simulink model "exampleModel_bus_axi_w_4ptavg"  (R2017b)
settings: Solver=VariableStepAuto  StartTime=0.0  StopTime=10e-5  RelTol=1e-3
PreLoadFcn:
  | setup
values from neighbouring files (symbols this model uses):
  axiClk = 156.25e6    (= 156250000)    [setup.m]    (also in setup_exampleModel_bus_axi_simulink.m; setup_exampleModel_bus_axi_simulink_lcls2.m; setup_lcls2_pcav.m; sysgen_signal.m)
  cav1p1_addr = 204    [setup_exampleModel_bus_axi_simulink.m]    (also in setup_exampleModel_bus_axi_simulink_lcls2.m; setup_lcls2_pcav.m; sysgen_signal.m)
  cav1p2_addr = cav1p1_addr * 2    (= 408)    [setup_exampleModel_bus_axi_simulink.m]    (also in setup_exampleModel_bus_axi_simulink_lcls2.m; setup_lcls2_pcav.m; sysgen_signal.m)
  cav2p1_addr = cav1p1_addr * 3    (= 612)    [setup_exampleModel_bus_axi_simulink.m]    (also in setup_exampleModel_bus_axi_simulink_lcls2.m; setup_lcls2_pcav.m; sysgen_signal.m)
  cav2p2_addr = cav1p1_addr * 4    (= 816)    [setup_exampleModel_bus_axi_simulink.m]    (also in setup_exampleModel_bus_axi_simulink_lcls2.m; setup_lcls2_pcav.m; sysgen_signal.m)
  Fadc = Fs/interleavedChannels    (= 29750000)    [setup.m]    (also in setup_exampleModel_bus_axi_simulink.m = 357000000; setup_exampleModel_bus_axi_simulink_lcls2.m = 351000000; setup_lcls2_pcav.m = 357000000; sysgen_signal.m = 357000000)
  fir_lpf = fir1(15, w_lpf)    [setup_exampleModel_bus_axi_simulink.m]    (also in setup_exampleModel_bus_axi_simulink_lcls2.m; setup_lcls2_pcav.m)
  Fproc = 204e6    (= 204000000)    [setup_exampleModel_bus_axi_simulink.m]    (also in setup_exampleModel_bus_axi_simulink_lcls2.m = 200571400; setup_lcls2_pcav.m; sysgen_signal.m)
  Fsig = Fproc/12    (= 17000000)    [setup_exampleModel_bus_axi_simulink.m]    (also in setup_exampleModel_bus_axi_simulink_lcls2.m = 16714283.3333; setup_lcls2_pcav.m)
  Tadc = 1/fadc    (= 2.80112044818e-09)    [cavity_signal.m]    (also in setup_exampleModel_bus_axi_simulink.m; setup_exampleModel_bus_axi_simulink_lcls2.m = 2.849002849e-09; setup_lcls2_pcav.m; setup_pcav_simulink.m)
undefined symbols (not defined in the file or in its folder): AXI4, Lite
libraries: xbsIndex_r4 x2870, llrf_lib x10, simulink x3
(part 10 of 15)

== system exampleModel_bus_axi_w_4ptavg/example/dsp/Cav2/c1p2_windowing_func3 ==
  imag : Inport
  real : Inport  Port=2
  eval_window : Inport  Port=3
  "CORDIC 6.0 " : xbsIndex_r4/CORDIC 6.0   functional_selection=Translate  architectural_configuration=Parallel  pipelining_mode=Maximum  data_format=SignedFraction  phase_format=Scaled_Radians  input_width=18  output_width=18  round_mode=Truncate  iterations=0  precision=0  compensation_scaling=No_Scale_Compensation  coarse_rotation=on  aclken=off  aresetn=off  out_tready=off  cartesian_has_tuser=off  cartesian_has_tlast=off  cartesian_tuser_width=1  phase_has_tuser=off  phase_has_tlast=off  phase_tuser_width=1  out_tlast_behv=Null  flow_control=NonBlocking  optimize_goal=Resources  trim_axipin_name=on  simulation_type=hybrid_sim  simulation_model=sysgen:cordic_v6_0  data_path_portlist={'s_axis_cartesian_tdata_imag', 's_axis_cartesian_tdata_real', 's_axis_phase_tdata_phase', 'm_axis_dout_tdata_imag', 'm_axis_dout_tdata_real', 'm_axis_dout_tdata_phase','m_axis_dout_tdata'}  ip_name=CORDIC  ip_version=6.0  dsptool_ready=true  ipcore_usecache=true  ipcore_useipmodelcache=true  wrapper_available=true  port_translation_map={ 'aclken' => 'en', 'aresetn' => 'rst' }  block_type=cordic_v6_0
      settings: infoedit=CORDIC 6.0
  Gateway Out{1..5,7} (6 alike) : xbsIndex_r4/Gateway Out  inherit_from_input=off  hdl_port=off  rows=1  columns=1  UseAsDAC=off  DACChannel='1'  interface=None  automatic_assignment=on  address_offset=hex2dec('00')  intf_name=''  intf_description=''  timing_constraint=None  locs_specified=off  LOCs={}  io_standard={}  block_type=gatewayout
  Scope{1..4} (4 alike) : Scope  NumInputPorts=3
  four_point_avg : Subsystem
  Window_profile : Outport
  wires:
  four_point_avg/1(Out1) -> Gateway Out2/1, Window_profile/1
  "CORDIC 6.0 "/3 -> Gateway Out4/1, Gateway Out1/1, four_point_avg/1(In1)
  [cav1_p2_dc_tvalid] -> "CORDIC 6.0 "/1
  imag/1 -> "CORDIC 6.0 "/2
  real/1 -> "CORDIC 6.0 "/3
  Gateway Out5/1 -> Scope3/1, Scope2/2
  Gateway Out7/1 -> Scope4/2, Scope3/2
  [c1p2_pt_cntr] -> Gateway Out7/1
  eval_window/1 -> [window]
  "CORDIC 6.0 "/2 -> Gateway Out5/1
  Gateway Out4/1 -> Scope4/1, Scope2/1
  Gateway Out1/1 -> Scope1/1
  Gateway Out2/1 -> Scope1/2
  [window] -> Gateway Out3/1
  Gateway Out3/1 -> Scope4/3

== system exampleModel_bus_axi_w_4ptavg/example/dsp/Cav2/c2p1_Masking_window1 ==
  note: delay for the comparison because Axilite register
      | takes a about 40 dsp clk cycles to load in
  phi_reset_trig : Inport
  start_pt : Inport  Port=2
  stop_pt : Inport  Port=3
  delay_amt : Inport  Port=4
  delay_latch : Inport  Port=5
  AddSub1 : xbsIndex_r4/AddSub  mode=Addition  use_carryin=off  use_carryout=off  en=off  latency=1  precision=User Defined  arith_type=Unsigned  n_bits=16  bin_pt=0  quantization=Truncate  overflow=Wrap  use_behavioral_HDL=off  hw_selection=Fabric  pipelined=off  dbl_ovrd=off  block_type=addsub
  AddSub4 : xbsIndex_r4/AddSub  mode=Addition  use_carryin=off  use_carryout=off  en=on  latency=1  precision=User Defined  arith_type=Unsigned  n_bits=16  bin_pt=0  quantization=Truncate  overflow=Saturate  use_behavioral_HDL=off  hw_selection=Fabric  pipelined=off  dbl_ovrd=off  block_type=addsub
  Constant1 : xbsIndex_r4/Constant  const=40  gui_display_data_type=Fixed-point  arith_type=Unsigned  n_bits=16  bin_pt=0  preci_type=Single  exp_width=8  frac_width=24  explicit_period=off  period=1  equ=P=C  opselect=C  inp2=PCIN>>17  opr=+  inp1=P  carry=CIN  dbl_ovrd=off  block_type=constant
  Constant11 : xbsIndex_r4/Constant  const=55  gui_display_data_type=Fixed-point  arith_type=Unsigned  n_bits=16  bin_pt=0  preci_type=Single  exp_width=8  frac_width=24  explicit_period=off  period=1  equ=P=C  opselect=C  inp2=PCIN>>17  opr=+  inp1=P  carry=CIN  dbl_ovrd=off  block_type=constant
  Constant2 : xbsIndex_r4/Constant  const=106  gui_display_data_type=Fixed-point  arith_type=Unsigned  n_bits=16  bin_pt=0  preci_type=Single  exp_width=8  frac_width=24  explicit_period=off  period=1  equ=P=C  opselect=C  inp2=PCIN>>17  opr=+  inp1=P  carry=CIN  dbl_ovrd=off  block_type=constant
  Constant3 : xbsIndex_r4/Constant  const=87  gui_display_data_type=Fixed-point  arith_type=Unsigned  n_bits=16  bin_pt=0  preci_type=Single  exp_width=8  frac_width=24  explicit_period=off  period=1  equ=P=C  opselect=C  inp2=PCIN>>17  opr=+  inp1=P  carry=CIN  dbl_ovrd=off  block_type=constant
  Convert{1,4..5,7..8} (5 alike) : xbsIndex_r4/Convert  gui_display_data_type=Boolean  arith_type=Boolean  n_bits=1  bin_pt=0  float_type=Single  exp_bits=8  fraction_bits=24  quantization=Truncate  overflow=Wrap  en=off  latency=1  pipeline=off  dbl_ovrd=off  block_type=convert
  Convert11 : xbsIndex_r4/Convert  gui_display_data_type=Fixed-point  arith_type=Unsigned  n_bits=1  bin_pt=0  float_type=Single  exp_bits=8  fraction_bits=24  quantization=Truncate  overflow=Wrap  en=off  latency=1  pipeline=off  dbl_ovrd=off  block_type=convert
  Convert2 : xbsIndex_r4/Convert  gui_display_data_type=Fixed-point  arith_type=Unsigned  n_bits=1  bin_pt=0  float_type=Single  exp_bits=8  fraction_bits=24  quantization=Truncate  overflow=Wrap  en=off  latency=1  pipeline=off  dbl_ovrd=off  block_type=convert
  Convert3 : xbsIndex_r4/Convert  gui_display_data_type=Boolean  arith_type=Boolean  n_bits=16  bin_pt=14  float_type=Single  exp_bits=8  fraction_bits=24  quantization=Truncate  overflow=Wrap  en=off  latency=1  pipeline=off  dbl_ovrd=off  block_type=convert
  Convert6 : xbsIndex_r4/Convert  gui_display_data_type=Fixed-point  arith_type=Unsigned  n_bits=8  bin_pt=0  float_type=Single  exp_bits=8  fraction_bits=24  quantization=Truncate  overflow=Saturate  en=off  latency=1  pipeline=off  dbl_ovrd=off  block_type=convert
  Counter : xbsIndex_r4/Counter  cnt_type=Count Limited  cnt_to=(2^15)  operation=Up  start_count=0  cnt_by_val=1  arith_type=Unsigned  n_bits=16  bin_pt=0  load_pin=off  rst=on  en=on  explicit_period=on  period=12/Fproc  use_behavioral_HDL=off  implementation=Fabric  dbl_ovrd=off  block_type=counter
  Delay{,1..4,6..7} (7 alike) : xbsIndex_r4/Delay  rst=off  infoeditControl=Selection of Reset will increase slice count due to use of real FFs and instead of SRLs  en=off  latency=1  reg_retiming=off  dbl_ovrd=off  block_type=delay
  Delay5 : xbsIndex_r4/Delay  rst=off  infoeditControl=Selection of Reset will increase slice count due to use of real FFs and instead of SRLs  en=off  latency=3  reg_retiming=off  dbl_ovrd=off  block_type=delay
  Display1 : Display
  Down Sample1 : xbsIndex_r4/Down Sample  sample_ratio=12  sample_phase="Last Value of Frame  (most efficient)"  en=off  rst=off  latency=1  dbl_ovrd=off  block_type=dsamp
  Down Sample2 : xbsIndex_r4/Down Sample  sample_ratio=12  sample_phase="Last Value of Frame  (most efficient)"  en=off  rst=off  latency=1  dbl_ovrd=off  block_type=dsamp
  Gateway Out{1..3,5,27..29} (7 alike) : xbsIndex_r4/Gateway Out  inherit_from_input=off  hdl_port=on  rows=1  columns=1  UseAsDAC=off  DACChannel='1'  interface=None  automatic_assignment=on  address_offset=hex2dec('00')  intf_name=''  intf_description=''  timing_constraint=None  locs_specified=off  LOCs={}  io_standard={}  block_type=gatewayout
  Gateway Out16 : xbsIndex_r4/Gateway Out  inherit_from_input=off  hdl_port=off  rows=1  columns=1  UseAsDAC=off  DACChannel='1'  interface=None  automatic_assignment=on  address_offset=hex2dec('00')  intf_name=''  intf_description=''  timing_constraint=None  locs_specified=off  LOCs={}  io_standard={}  block_type=gatewayout
  Gateway Out17 : xbsIndex_r4/Gateway Out  inherit_from_input=off  hdl_port=off  rows=1  columns=1  UseAsDAC=off  DACChannel='1'  interface=None  automatic_assignment=on  address_offset=hex2dec('00')  intf_name=''  intf_description=''  timing_constraint=None  locs_specified=off  LOCs={}  io_standard={}  block_type=gatewayout
  Gateway Out18 : xbsIndex_r4/Gateway Out  inherit_from_input=off  hdl_port=off  rows=1  columns=1  UseAsDAC=off  DACChannel='1'  interface=None  automatic_assignment=on  address_offset=hex2dec('00')  intf_name=''  intf_description=''  timing_constraint=None  locs_specified=off  LOCs={}  io_standard={}  block_type=gatewayout
  Logical1 : xbsIndex_r4/Logical  logical_function=AND  inputs=2  en=off  latency=1  precision=Full  arith_type=Unsigned  n_bits=16  bin_pt=0  align_bp=on  dbl_ovrd=off  block_type=logical
  Logical2 : xbsIndex_r4/Logical  logical_function=AND  inputs=2  en=off  latency=1  precision=Full  arith_type=Unsigned  n_bits=16  bin_pt=0  align_bp=on  dbl_ovrd=off  block_type=logical
  Register : xbsIndex_r4/Register  init=44  rst=off  en=on  dbl_ovrd=off  block_type=register
  Register1 : xbsIndex_r4/Register  init=0  rst=off  en=on  dbl_ovrd=off  block_type=register
  Register10 : xbsIndex_r4/Register  init=0  rst=off  en=off  dbl_ovrd=off  block_type=register
  Register5 : xbsIndex_r4/Register  init=0  rst=off  en=off  dbl_ovrd=off  block_type=register
  Register6 : xbsIndex_r4/Register  init=100  rst=off  en=off  dbl_ovrd=off  block_type=register
  Relational1 : xbsIndex_r4/Relational  mode=a<b  op_type=Bool  en=on  latency=1  dbl_ovrd=off  block_type=relational
  Relational2 : xbsIndex_r4/Relational  mode=a>b  op_type=Bool  en=off  latency=1  dbl_ovrd=off  block_type=relational
  Relational3 : xbsIndex_r4/Relational  mode=a<b  op_type=Bool  en=on  latency=1  dbl_ovrd=off  block_type=relational
  Relational4 : xbsIndex_r4/Relational  mode=a>b  op_type=Bool  en=on  latency=1  dbl_ovrd=off  block_type=relational
  Relational5 : xbsIndex_r4/Relational  mode=a<b  op_type=Bool  en=on  latency=1  dbl_ovrd=off  block_type=relational
  Relational6 : xbsIndex_r4/Relational  mode=a>b  op_type=Bool  en=on  latency=1  dbl_ovrd=off  block_type=relational
  Scope1 : Scope  NumInputPorts=3
  Scope10 : Scope  NumInputPorts=3
  Scope2 : Scope  NumInputPorts=2
  Scope5 : Scope  NumInputPorts=3
  counter : Outport
  eval_window : Outport  Port=2
  integral_trig : Outport  Port=3
  flo_window : Outport  Port=4
  delay_val : Outport  Port=5
  wires:
  Gateway Out5/1 -> Scope2/2
  start_pt/1 -> Register5/1
  phi_reset_trig/1 -> Register10/1
  Register5/1 -> Down Sample1/1
  stop_pt/1 -> Register6/1
  Register6/1 -> Down Sample2/1
  Delay2/1 -> Relational4/2
  Delay3/1 -> AddSub1/1, Gateway Out2/1, Relational3/2
  Constant1/1 -> Relational2/2
  Relational3/1 -> Gateway Out28/1, Convert7/1
  Relational4/1 -> Gateway Out27/1, Convert8/1
  Gateway Out28/1 -> Scope10/2
  Gateway Out29/1 -> Scope2/1, Scope10/3
  Gateway Out27/1 -> Scope10/1
  Logical1/1 -> Convert11/1
  Convert8/1 -> Logical1/1
  Convert7/1 -> Gateway Out3/1, Logical1/2
  Convert11/1 -> eval_window/1, Gateway Out29/1
  Convert5/1 -> integral_trig/1, Gateway Out5/1
  Relational5/1 -> Convert5/1
  Relational2/1 -> Relational6/3, Relational1/3, Relational5/3, Relational3/3, Relational4/3
  Counter/1 -> Convert6/1
  Constant11/1 -> AddSub1/2
  AddSub1/1 -> Relational5/2
  Register10/1 -> Convert3/1
  Down Sample1/1 -> Delay2/1
  Down Sample2/1 -> Delay3/1
  Gateway Out1/1 -> Scope1/1
  Gateway Out2/1 -> Scope1/2
  Gateway Out3/1 -> Scope1/3
  Delay1/1 -> Relational4/1
  Delay4/1 -> Relational3/1
  Delay5/1 -> Gateway Out1/1
  Delay7/1 -> Relational1/1
  Constant2/1 -> Relational1/2
  Relational1/1 -> Convert1/1
  Logical2/1 -> Convert2/1
  Convert1/1 -> Logical2/2
  Convert2/1 -> flo_window/1
  Delay6/1 -> Relational6/1
  Constant3/1 -> Relational6/2
  Relational6/1 -> Convert4/1
  Convert4/1 -> Logical2/1
  Gateway Out18/1 -> Scope5/3
  delay_latch/1 -> Gateway Out18/1, Delay/1, AddSub4/3
  Register/1 -> AddSub4/1, delay_val/1, Gateway Out17/1
  Delay/1 -> Register/2
  Gateway Out17/1 -> Scope5/2
  delay_amt/1 -> AddSub4/2, Gateway Out16/1
  Gateway Out16/1 -> Scope5/1, Display1/1
  AddSub4/1 -> Register/1
  Convert3/1 -> Register1/2, Register1/1, Counter/1
  Register1/1 -> Counter/2
  Convert6/1 -> Delay5/1, counter/1, Delay1/1, Delay4/1, Relational2/1, Delay6/1, Delay7/1, Relational5/1

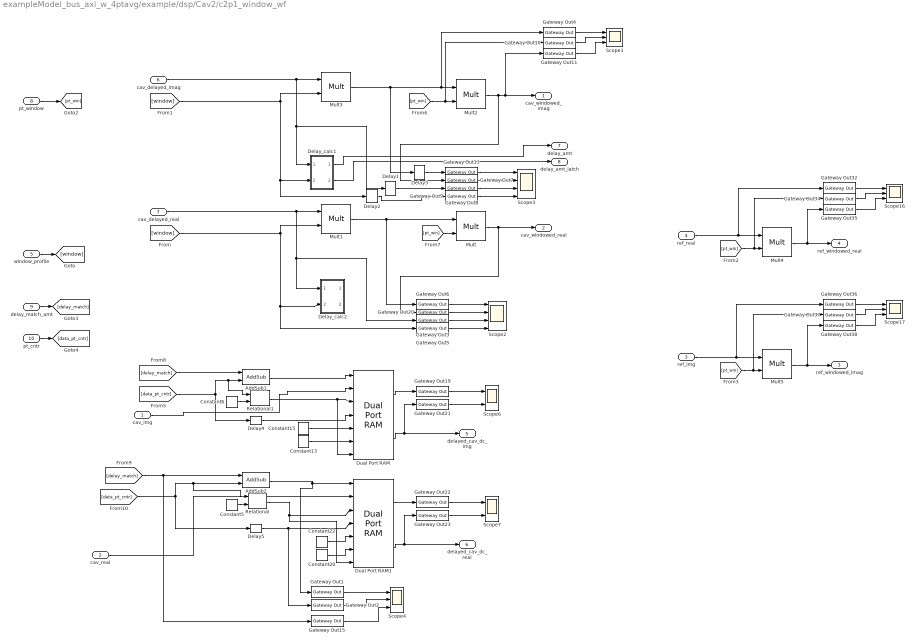
== system exampleModel_bus_axi_w_4ptavg/example/dsp/Cav2/c2p1_window_wf  ==
  cav_img : Inport
  cav_real : Inport  Port=2
  ref_img : Inport  Port=3
  ref_real : Inport  Port=4
  window_profile : Inport  Port=5
  cav_delayed_imag : Inport  Port=6
  cav_delayed_real : Inport  Port=7
  pt_window : Inport  Port=8
  delay_match_amt : Inport  Port=9
  pt_cntr : Inport  Port=10
  AddSub1 : xbsIndex_r4/AddSub  mode=Addition  use_carryin=off  use_carryout=off  en=off  latency=1  precision=User Defined  arith_type=Unsigned  n_bits=16  bin_pt=0  quantization=Truncate  overflow=Wrap  use_behavioral_HDL=off  hw_selection=Fabric  pipelined=off  dbl_ovrd=off  block_type=addsub
  AddSub2 : xbsIndex_r4/AddSub  mode=Addition  use_carryin=off  use_carryout=off  en=off  latency=1  precision=User Defined  arith_type=Unsigned  n_bits=16  bin_pt=0  quantization=Truncate  overflow=Wrap  use_behavioral_HDL=off  hw_selection=Fabric  pipelined=off  dbl_ovrd=off  block_type=addsub
  Constant13 : xbsIndex_r4/Constant  const=1  gui_display_data_type=Boolean  arith_type=Boolean  n_bits=16  bin_pt=14  preci_type=Single  exp_width=8  frac_width=24  explicit_period=off  period=1  equ=P=C  opselect=C  inp2=PCIN>>17  opr=+  inp1=P  carry=CIN  dbl_ovrd=off  block_type=constant
  Constant{5..6,15,22} (4 alike) : xbsIndex_r4/Constant  const=0  gui_display_data_type=Fixed-point  arith_type=Signed (2's comp)  n_bits=18  bin_pt=16  preci_type=Single  exp_width=8  frac_width=24  explicit_period=off  period=1  equ=P=C  opselect=C  inp2=PCIN>>17  opr=+  inp1=P  carry=CIN  dbl_ovrd=off  block_type=constant
  Constant20 : xbsIndex_r4/Constant  const=1  gui_display_data_type=Boolean  arith_type=Boolean  n_bits=16  bin_pt=14  preci_type=Single  exp_width=8  frac_width=24  explicit_period=off  period=1  equ=P=C  opselect=C  inp2=PCIN>>17  opr=+  inp1=P  carry=CIN  dbl_ovrd=off  block_type=constant
  Delay1 : xbsIndex_r4/Delay  rst=off  infoeditControl=Selection of Reset will increase slice count due to use of real FFs and instead of SRLs  en=off  latency=6  reg_retiming=off  dbl_ovrd=off  block_type=delay
  Delay2 : xbsIndex_r4/Delay  rst=off  infoeditControl=Selection of Reset will increase slice count due to use of real FFs and instead of SRLs  en=off  latency=6  reg_retiming=off  dbl_ovrd=off  block_type=delay
  Delay3 : xbsIndex_r4/Delay  rst=off  infoeditControl=Selection of Reset will increase slice count due to use of real FFs and instead of SRLs  en=off  latency=3  reg_retiming=off  dbl_ovrd=off  block_type=delay
  Delay4 : xbsIndex_r4/Delay  rst=off  infoeditControl=Selection of Reset will increase slice count due to use of real FFs and instead of SRLs  en=off  latency=1  reg_retiming=off  dbl_ovrd=off  block_type=delay
  Delay5 : xbsIndex_r4/Delay  rst=off  infoeditControl=Selection of Reset will increase slice count due to use of real FFs and instead of SRLs  en=off  latency=1  reg_retiming=off  dbl_ovrd=off  block_type=delay
  Delay_calc1 : Subsystem
  Delay_calc2 : Subsystem
  Dual Port RAM : xbsIndex_r4/Dual Port RAM  depth=2^16  initVector=zeros(2^16,1)  distributed_mem=Block RAM  init_a=0  init_b=0  rst_a=off  rst_b=off  en_a=off  en_b=on  latency=1  write_mode_A=Read After Write  write_mode_B=Read Before Write  optimize=Area  dbl_ovrd=off  block_type=dpram
  Dual Port RAM1 : xbsIndex_r4/Dual Port RAM  depth=2^16  initVector=zeros(2^16,1)  distributed_mem=Block RAM  init_a=0  init_b=0  rst_a=off  rst_b=off  en_a=off  en_b=on  latency=1  write_mode_A=Read After Write  write_mode_B=Read Before Write  optimize=Area  dbl_ovrd=off  block_type=dpram
  Gateway Out{1..3,5..9,13,15,19..23} (15 alike) : xbsIndex_r4/Gateway Out  inherit_from_input=off  hdl_port=off  rows=1  columns=1  UseAsDAC=off  DACChannel='1'  interface=None  automatic_assignment=on  address_offset=hex2dec('00')  intf_name=''  intf_description=''  timing_constraint=None  locs_specified=off  LOCs={}  io_standard={}  block_type=gatewayout
  Gateway Out{4,10..11,32,34..38} (9 alike) : xbsIndex_r4/Gateway Out  inherit_from_input=off  hdl_port=on  rows=1  columns=1  UseAsDAC=off  DACChannel='1'  interface=None  automatic_assignment=on  address_offset=hex2dec('00')  intf_name=''  intf_description=''  timing_constraint=None  locs_specified=off  LOCs={}  io_standard={}  block_type=gatewayout
  Mult{,2,4..5} (4 alike) : xbsIndex_r4/Mult  precision=User Defined  arith_type="Signed  (2's comp)"  n_bits=18  bin_pt=16  quantization=Truncate  overflow=Wrap  en=off  latency=3  use_behavioral_HDL=off  opt=Speed  use_embedded=on  optimum_pipeline=off  pipeline=on  dbl_ovrd=off  use_rpm=on  placement_style=Triangular  block_type=mult
  Mult1 : xbsIndex_r4/Mult  precision=User Defined  arith_type="Signed  (2's comp)"  n_bits=18  bin_pt=17  quantization=Truncate  overflow=Wrap  en=off  latency=3  use_behavioral_HDL=off  opt=Speed  use_embedded=on  optimum_pipeline=off  pipeline=on  dbl_ovrd=off  use_rpm=on  placement_style=Triangular  block_type=mult
  Mult3 : xbsIndex_r4/Mult  precision=User Defined  arith_type="Signed  (2's comp)"  n_bits=18  bin_pt=17  quantization=Truncate  overflow=Wrap  en=off  latency=3  use_behavioral_HDL=off  opt=Speed  use_embedded=on  optimum_pipeline=off  pipeline=on  dbl_ovrd=off  use_rpm=on  placement_style=Triangular  block_type=mult
  Relational : xbsIndex_r4/Relational  mode=a>b  op_type=Bool  en=off  latency=1  dbl_ovrd=off  block_type=relational
  Relational1 : xbsIndex_r4/Relational  mode=a>b  op_type=Bool  en=off  latency=1  dbl_ovrd=off  block_type=relational
  Scope{1,4,16..17} (4 alike) : Scope  NumInputPorts=3
  Scope2 : Scope  NumInputPorts=4
  Scope3 : Scope  NumInputPorts=4
  Scope6 : Scope  NumInputPorts=2
  Scope7 : Scope  NumInputPorts=2
  cav_windowed_imag : Outport
  cav_windowed_real : Outport  Port=2
  ref_windowed_imag : Outport  Port=3
  ref_windowed_real : Outport  Port=4
  delayed_cav_dc_img : Outport  Port=5
  delayed_cav_dc_real : Outport  Port=6
  delay_amt : Outport  Port=7
  delay_amt_latch : Outport  Port=8
  wires:
  cav_real/1 -> Dual Port RAM1/2
  Relational/1 -> Dual Port RAM1/7, Dual Port RAM1/3
  Mult2/1 -> Gateway Out11/1, cav_windowed_imag/1, Gateway Out7/1
  Gateway Out23/1 -> Scope7/2
  Gateway Out21/1 -> Scope6/2
  Dual Port RAM1/1 -> Gateway Out22/1
  [data_pt_cntr] -> Relational1/1, AddSub1/2, Delay4/1
  Constant15/1 -> Dual Port RAM/5
  Gateway Out20/1 -> Scope2/2
  AddSub1/1 -> Dual Port RAM/1
  [pt_win] -> Gateway Out10/1, Mult2/2
  Gateway Out8/1 -> Scope3/3
  Gateway Out3/1 -> Scope2/3
  Constant13/1 -> Dual Port RAM/6
  Mult/1 -> cav_windowed_real/1, Gateway Out20/1
  cav_delayed_imag/1 -> Mult3/1, Delay_calc1/1(wav), Delay1/1
  [delay_match] -> Gateway Out15/1, AddSub2/1
  Gateway Out19/1 -> Scope6/1
  Gateway Out9/1 -> Scope3/4
  [data_pt_cntr] -> Delay5/1, Relational/1, AddSub2/2
  Dual Port RAM/1 -> Gateway Out19/1
  Gateway Out22/1 -> Scope7/1
  [window] -> Delay_calc1/2(win), Delay2/1, Mult3/2
  [window] -> Mult1/2, Delay_calc2/2(win), Gateway Out5/1
  cav_delayed_real/1 -> Delay_calc2/1(wav), Gateway Out3/1, Mult1/1
  Constant20/1 -> Dual Port RAM1/6
  Mult1/1 -> Gateway Out6/1, Mult/1
  Constant22/1 -> Dual Port RAM1/5
  Gateway Out6/1 -> Scope2/1
  Gateway Out13/1 -> Scope3/1
  [delay_match] -> AddSub1/1
  Gateway Out5/1 -> Scope2/4
  Gateway Out7/1 -> Scope3/2
  [pt_win] -> Mult/2
  Gateway Out35/1 -> Scope16/3
  ref_img/1 -> Gateway Out36/1, Mult5/1
  [pt_win] -> Gateway Out37/1, Mult5/2
  [pt_win] -> Gateway Out34/1, Mult4/2
  ref_real/1 -> Gateway Out32/1, Mult4/1
  Mult5/1 -> ref_windowed_imag/1, Gateway Out38/1
  Gateway Out38/1 -> Scope17/3
  Gateway Out36/1 -> Scope17/1
  Gateway Out32/1 -> Scope16/1
  Gateway Out34/1 -> Scope16/2
  Mult4/1 -> ref_windowed_real/1, Gateway Out35/1
  Gateway Out37/1 -> Scope17/2
  window_profile/1 -> [window]
  Delay_calc1/1(delay_amt) -> delay_amt/1
  pt_window/1 -> [pt_win]
  delay_match_amt/1 -> [delay_match]
  pt_cntr/1 -> [data_pt_cntr]
  Mult3/1 -> Delay3/1, Gateway Out4/1, Mult2/1
  Delay1/1 -> Gateway Out8/1
  Delay2/1 -> Gateway Out9/1
  Delay3/1 -> Gateway Out13/1
  Delay_calc1/2(delay_fb_latch) -> delay_amt_latch/1
  Gateway Out1/1 -> Scope4/1
  Gateway Out2/1 -> Scope4/2
  AddSub2/1 -> Gateway Out1/1, Dual Port RAM1/1
  cav_img/1 -> Dual Port RAM/2
  Delay4/1 -> Dual Port RAM/4
  Gateway Out15/1 -> Scope4/3
  Delay5/1 -> Gateway Out2/1, Dual Port RAM1/4
  Dual Port RAM1/2 -> delayed_cav_dc_real/1, Gateway Out23/1
  Dual Port RAM/2 -> delayed_cav_dc_img/1, Gateway Out21/1
  Constant5/1 -> Relational/2
  Constant6/1 -> Relational1/2
  Relational1/1 -> Dual Port RAM/7, Dual Port RAM/3
  Gateway Out10/1 -> Scope1/2
  Gateway Out4/1 -> Scope1/1
  Gateway Out11/1 -> Scope1/3

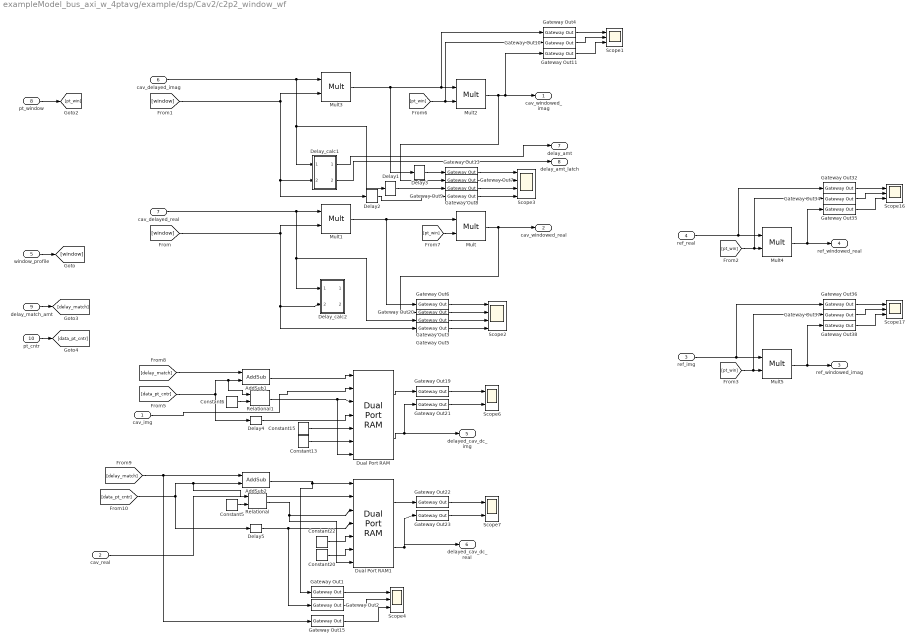
== system exampleModel_bus_axi_w_4ptavg/example/dsp/Cav2/c2p2_window_wf ==
  cav_img : Inport
  cav_real : Inport  Port=2
  ref_img : Inport  Port=3
  ref_real : Inport  Port=4
  window_profile : Inport  Port=5
  cav_delayed_imag : Inport  Port=6
  cav_delayed_real : Inport  Port=7
  pt_window : Inport  Port=8
  delay_match_amt : Inport  Port=9
  pt_cntr : Inport  Port=10
  AddSub1 : xbsIndex_r4/AddSub  mode=Addition  use_carryin=off  use_carryout=off  en=off  latency=1  precision=User Defined  arith_type=Unsigned  n_bits=16  bin_pt=0  quantization=Truncate  overflow=Wrap  use_behavioral_HDL=off  hw_selection=Fabric  pipelined=off  dbl_ovrd=off  block_type=addsub
  AddSub2 : xbsIndex_r4/AddSub  mode=Addition  use_carryin=off  use_carryout=off  en=off  latency=1  precision=User Defined  arith_type=Unsigned  n_bits=16  bin_pt=0  quantization=Truncate  overflow=Wrap  use_behavioral_HDL=off  hw_selection=Fabric  pipelined=off  dbl_ovrd=off  block_type=addsub
  Constant13 : xbsIndex_r4/Constant  const=1  gui_display_data_type=Boolean  arith_type=Boolean  n_bits=16  bin_pt=14  preci_type=Single  exp_width=8  frac_width=24  explicit_period=off  period=1  equ=P=C  opselect=C  inp2=PCIN>>17  opr=+  inp1=P  carry=CIN  dbl_ovrd=off  block_type=constant
  Constant{5..6,15,22} (4 alike) : xbsIndex_r4/Constant  const=0  gui_display_data_type=Fixed-point  arith_type=Signed (2's comp)  n_bits=18  bin_pt=16  preci_type=Single  exp_width=8  frac_width=24  explicit_period=off  period=1  equ=P=C  opselect=C  inp2=PCIN>>17  opr=+  inp1=P  carry=CIN  dbl_ovrd=off  block_type=constant
  Constant20 : xbsIndex_r4/Constant  const=1  gui_display_data_type=Boolean  arith_type=Boolean  n_bits=16  bin_pt=14  preci_type=Single  exp_width=8  frac_width=24  explicit_period=off  period=1  equ=P=C  opselect=C  inp2=PCIN>>17  opr=+  inp1=P  carry=CIN  dbl_ovrd=off  block_type=constant
  Delay1 : xbsIndex_r4/Delay  rst=off  infoeditControl=Selection of Reset will increase slice count due to use of real FFs and instead of SRLs  en=off  latency=6  reg_retiming=off  dbl_ovrd=off  block_type=delay
  Delay2 : xbsIndex_r4/Delay  rst=off  infoeditControl=Selection of Reset will increase slice count due to use of real FFs and instead of SRLs  en=off  latency=6  reg_retiming=off  dbl_ovrd=off  block_type=delay
  Delay3 : xbsIndex_r4/Delay  rst=off  infoeditControl=Selection of Reset will increase slice count due to use of real FFs and instead of SRLs  en=off  latency=3  reg_retiming=off  dbl_ovrd=off  block_type=delay
  Delay4 : xbsIndex_r4/Delay  rst=off  infoeditControl=Selection of Reset will increase slice count due to use of real FFs and instead of SRLs  en=off  latency=1  reg_retiming=off  dbl_ovrd=off  block_type=delay
  Delay5 : xbsIndex_r4/Delay  rst=off  infoeditControl=Selection of Reset will increase slice count due to use of real FFs and instead of SRLs  en=off  latency=1  reg_retiming=off  dbl_ovrd=off  block_type=delay
  Delay_calc1 : Subsystem
  Delay_calc2 : Subsystem
  Dual Port RAM : xbsIndex_r4/Dual Port RAM  depth=2^16  initVector=zeros(2^16,1)  distributed_mem=Block RAM  init_a=0  init_b=0  rst_a=off  rst_b=off  en_a=off  en_b=on  latency=1  write_mode_A=Read After Write  write_mode_B=Read Before Write  optimize=Area  dbl_ovrd=off  block_type=dpram
  Dual Port RAM1 : xbsIndex_r4/Dual Port RAM  depth=2^16  initVector=zeros(2^16,1)  distributed_mem=Block RAM  init_a=0  init_b=0  rst_a=off  rst_b=off  en_a=off  en_b=on  latency=1  write_mode_A=Read After Write  write_mode_B=Read Before Write  optimize=Area  dbl_ovrd=off  block_type=dpram
  Gateway Out{1..3,5..9,13,15,19..23} (15 alike) : xbsIndex_r4/Gateway Out  inherit_from_input=off  hdl_port=off  rows=1  columns=1  UseAsDAC=off  DACChannel='1'  interface=None  automatic_assignment=on  address_offset=hex2dec('00')  intf_name=''  intf_description=''  timing_constraint=None  locs_specified=off  LOCs={}  io_standard={}  block_type=gatewayout
  Gateway Out{4,10..11,32,34..38} (9 alike) : xbsIndex_r4/Gateway Out  inherit_from_input=off  hdl_port=on  rows=1  columns=1  UseAsDAC=off  DACChannel='1'  interface=None  automatic_assignment=on  address_offset=hex2dec('00')  intf_name=''  intf_description=''  timing_constraint=None  locs_specified=off  LOCs={}  io_standard={}  block_type=gatewayout
  Mult{,2,4..5} (4 alike) : xbsIndex_r4/Mult  precision=User Defined  arith_type="Signed  (2's comp)"  n_bits=18  bin_pt=16  quantization=Truncate  overflow=Wrap  en=off  latency=3  use_behavioral_HDL=off  opt=Speed  use_embedded=on  optimum_pipeline=off  pipeline=on  dbl_ovrd=off  use_rpm=on  placement_style=Triangular  block_type=mult
  Mult1 : xbsIndex_r4/Mult  precision=User Defined  arith_type="Signed  (2's comp)"  n_bits=18  bin_pt=17  quantization=Truncate  overflow=Wrap  en=off  latency=3  use_behavioral_HDL=off  opt=Speed  use_embedded=on  optimum_pipeline=off  pipeline=on  dbl_ovrd=off  use_rpm=on  placement_style=Triangular  block_type=mult
  Mult3 : xbsIndex_r4/Mult  precision=User Defined  arith_type="Signed  (2's comp)"  n_bits=18  bin_pt=17  quantization=Truncate  overflow=Wrap  en=off  latency=3  use_behavioral_HDL=off  opt=Speed  use_embedded=on  optimum_pipeline=off  pipeline=on  dbl_ovrd=off  use_rpm=on  placement_style=Triangular  block_type=mult
  Relational : xbsIndex_r4/Relational  mode=a>b  op_type=Bool  en=off  latency=1  dbl_ovrd=off  block_type=relational
  Relational1 : xbsIndex_r4/Relational  mode=a>b  op_type=Bool  en=off  latency=1  dbl_ovrd=off  block_type=relational
  Scope{1,4,16..17} (4 alike) : Scope  NumInputPorts=3
  Scope2 : Scope  NumInputPorts=4
  Scope3 : Scope  NumInputPorts=4
  Scope6 : Scope  NumInputPorts=2
  Scope7 : Scope  NumInputPorts=2
  cav_windowed_imag : Outport
  cav_windowed_real : Outport  Port=2
  ref_windowed_imag : Outport  Port=3
  ref_windowed_real : Outport  Port=4
  delayed_cav_dc_img : Outport  Port=5
  delayed_cav_dc_real : Outport  Port=6
  delay_amt : Outport  Port=7
  delay_amt_latch : Outport  Port=8
  wires:
  cav_real/1 -> Dual Port RAM1/2
  Relational/1 -> Dual Port RAM1/7, Dual Port RAM1/3
  Mult2/1 -> Gateway Out11/1, cav_windowed_imag/1, Gateway Out7/1
  Gateway Out23/1 -> Scope7/2
  Gateway Out21/1 -> Scope6/2
  Dual Port RAM1/1 -> Gateway Out22/1
  [data_pt_cntr] -> Relational1/1, AddSub1/2, Delay4/1
  Constant15/1 -> Dual Port RAM/5
  Gateway Out20/1 -> Scope2/2
  AddSub1/1 -> Dual Port RAM/1
  [pt_win] -> Gateway Out10/1, Mult2/2
  Gateway Out8/1 -> Scope3/3
  Gateway Out3/1 -> Scope2/3
  Constant13/1 -> Dual Port RAM/6
  Mult/1 -> cav_windowed_real/1, Gateway Out20/1
  cav_delayed_imag/1 -> Mult3/1, Delay_calc1/1(wav), Delay1/1
  [delay_match] -> Gateway Out15/1, AddSub2/1
  Gateway Out19/1 -> Scope6/1
  Gateway Out9/1 -> Scope3/4
  [data_pt_cntr] -> Delay5/1, Relational/1, AddSub2/2
  Dual Port RAM/1 -> Gateway Out19/1
  Gateway Out22/1 -> Scope7/1
  [window] -> Delay_calc1/2(win), Delay2/1, Mult3/2
  [window] -> Mult1/2, Delay_calc2/2(win), Gateway Out5/1
  cav_delayed_real/1 -> Delay_calc2/1(wav), Gateway Out3/1, Mult1/1
  Constant20/1 -> Dual Port RAM1/6
  Mult1/1 -> Gateway Out6/1, Mult/1
  Constant22/1 -> Dual Port RAM1/5
  Gateway Out6/1 -> Scope2/1
  Gateway Out13/1 -> Scope3/1
  [delay_match] -> AddSub1/1
  Gateway Out5/1 -> Scope2/4
  Gateway Out7/1 -> Scope3/2
  [pt_win] -> Mult/2
  Gateway Out35/1 -> Scope16/3
  ref_img/1 -> Gateway Out36/1, Mult5/1
  [pt_win] -> Gateway Out37/1, Mult5/2
  [pt_win] -> Gateway Out34/1, Mult4/2
  ref_real/1 -> Gateway Out32/1, Mult4/1
  Mult5/1 -> ref_windowed_imag/1, Gateway Out38/1
  Gateway Out38/1 -> Scope17/3
  Gateway Out36/1 -> Scope17/1
  Gateway Out32/1 -> Scope16/1
  Gateway Out34/1 -> Scope16/2
  Mult4/1 -> ref_windowed_real/1, Gateway Out35/1
  Gateway Out37/1 -> Scope17/2
  window_profile/1 -> [window]
  Delay_calc1/1(delay_amt) -> delay_amt/1
  pt_window/1 -> [pt_win]
  delay_match_amt/1 -> [delay_match]
  pt_cntr/1 -> [data_pt_cntr]
  Mult3/1 -> Delay3/1, Gateway Out4/1, Mult2/1
  Delay1/1 -> Gateway Out8/1
  Delay2/1 -> Gateway Out9/1
  Delay3/1 -> Gateway Out13/1
  Delay_calc1/2(delay_fb_latch) -> delay_amt_latch/1
  Gateway Out1/1 -> Scope4/1
  Gateway Out2/1 -> Scope4/2
  AddSub2/1 -> Gateway Out1/1, Dual Port RAM1/1
  cav_img/1 -> Dual Port RAM/2
  Delay4/1 -> Dual Port RAM/4
  Gateway Out15/1 -> Scope4/3
  Delay5/1 -> Gateway Out2/1, Dual Port RAM1/4
  Dual Port RAM1/2 -> delayed_cav_dc_real/1, Gateway Out23/1
  Dual Port RAM/2 -> delayed_cav_dc_img/1, Gateway Out21/1
  Constant5/1 -> Relational/2
  Constant6/1 -> Relational1/2
  Relational1/1 -> Dual Port RAM/7, Dual Port RAM/3
  Gateway Out10/1 -> Scope1/2
  Gateway Out4/1 -> Scope1/1
  Gateway Out11/1 -> Scope1/3

== system exampleModel_bus_axi_w_4ptavg/example/dsp/Ref/IQ_select ==
  IQ_stream_in : Inport
  IQ_chan_sel : Inport  Port=2
  Bus Creator5 : BusCreator  Inputs=3
  Bus Selector : BusSelector  OutputSignals=ddcI,ddcQ,sync
  Bus Selector3 : BusSelector  OutputSignals=ddcI,ddcQ,ddcSync,ddcChannel
  Channel Select3 : llrf_lib/Sysgen/Single Rate/Channel Select  SystemSampleTime=-1
      settings: SourceProductName=LLRF Library
  ddcI : Outport
  ddcQ : Outport  Port=2
  sync : Outport  Port=3
  wires:
  IQ_stream_in/1 -> Bus Selector3/1
  IQ_chan_sel/1 -> Channel Select3/5
  Channel Select3/3 -> Bus Creator5/3  "sync"
  Bus Selector3/2 -> Channel Select3/2  "<ddcQ>"
  Channel Select3/1 -> Bus Creator5/1  "ddcI"
  Channel Select3/2 -> Bus Creator5/2  "ddcQ"
  Bus Selector3/1 -> Channel Select3/1  "<ddcI>"
  Bus Selector3/4 -> Channel Select3/4  "<ddcChannel>"
  Bus Selector3/3 -> Channel Select3/3  "<ddcSync>"
  Bus Creator5/1 -> Bus Selector/1
  Bus Selector/1 -> ddcI/1  "<ddcI>"
  Bus Selector/2 -> ddcQ/1  "<ddcQ>"
  Bus Selector/3 -> sync/1  "<sync>"

== system exampleModel_bus_axi_w_4ptavg/example/dsp/Ref/PA_select ==
  PA_bus : Inport
  PA_chan_sel : Inport  Port=2
  Bus Selector1 : BusSelector  OutputSignals=amp,phase,sync,channel
  Channel Select1 : llrf_lib/Sysgen/Single Rate/Channel Select  SystemSampleTime=-1
      settings: SourceProductName=LLRF Library
  Amp : Outport
  Phase : Outport  Port=2
  sync : Outport  Port=3
  wires:
  PA_bus/1 -> Bus Selector1/1
  PA_chan_sel/1 -> Channel Select1/5
  Channel Select1/3 -> sync/1  "sync"
  Channel Select1/2 -> Phase/1  "phase"
  Channel Select1/1 -> Amp/1  "amp"
  Bus Selector1/4 -> Channel Select1/4  "<channel>"
  Bus Selector1/3 -> Channel Select1/3  "<sync>"
  Bus Selector1/2 -> Channel Select1/2  "<phase>"
  Bus Selector1/1 -> Channel Select1/1  "<amp>"

== system exampleModel_bus_axi_w_4ptavg/example/dsp/Cav1/DDC NCO1/pulse_catcher ==
  In1 : Inport
  Convert : xbsIndex_r4/Convert  gui_display_data_type=Boolean  arith_type=Boolean  n_bits=16  bin_pt=14  float_type=Single  exp_bits=8  fraction_bits=24  quantization=Truncate  overflow=Wrap  en=off  latency=1  pipeline=off  dbl_ovrd=off  block_type=convert
  Delay : xbsIndex_r4/Delay  rst=off  infoeditControl=Selection of Reset will increase slice count due to use of real FFs and instead of SRLs  en=off  latency=5  reg_retiming=off  dbl_ovrd=off  block_type=delay
  Delay1 : xbsIndex_r4/Delay  rst=off  infoeditControl=Selection of Reset will increase slice count due to use of real FFs and instead of SRLs  en=off  latency=1  reg_retiming=off  dbl_ovrd=off  block_type=delay
  Register : xbsIndex_r4/Register  init=0  rst=on  en=on  dbl_ovrd=off  block_type=register
  Out1 : Outport
  wires:
  In1/1 -> Convert/1, Delay1/1
  Delay/1 -> Register/2
  Register/1 -> Out1/1
  Convert/1 -> Register/3, Delay/1
  Delay1/1 -> Register/1

== system exampleModel_bus_axi_w_4ptavg/example/dsp/Cav1/Subsystem/four_point_avg ==
  In1 : Inport
  AddSub1 : xbsIndex_r4/AddSub  mode=Addition  use_carryin=off  use_carryout=off  en=off  latency=1  precision=User Defined  arith_type="Signed  (2's comp)"  n_bits=33  bin_pt=31  quantization=Truncate  overflow=Saturate  use_behavioral_HDL=off  hw_selection=Fabric  pipelined=off  dbl_ovrd=off  block_type=addsub
  AddSub2 : xbsIndex_r4/AddSub  mode=Addition  use_carryin=off  use_carryout=off  en=off  latency=1  precision=User Defined  arith_type="Signed  (2's comp)"  n_bits=33  bin_pt=31  quantization=Truncate  overflow=Saturate  use_behavioral_HDL=off  hw_selection=Fabric  pipelined=off  dbl_ovrd=off  block_type=addsub
  AddSub3 : xbsIndex_r4/AddSub  mode=Addition  use_carryin=off  use_carryout=off  en=off  latency=1  precision=User Defined  arith_type="Signed  (2's comp)"  n_bits=33  bin_pt=31  quantization=Truncate  overflow=Saturate  use_behavioral_HDL=off  hw_selection=Fabric  pipelined=off  dbl_ovrd=off  block_type=addsub
  CMult{1..4} (4 alike) : xbsIndex_r4/CMult  const=0.25  gui_display_data_type=Fixed-point  const_n_bits=18  const_bin_pt=16  float_type=Single  exp_bits=8  fraction_bits=24  en=off  latency=1  precision=User Defined  arith_type="Signed  (2's comp)"  n_bits=33  bin_pt=31  quantization=Truncate  overflow=Saturate  use_behavioral_HDL=off  mem_type=Distributed RAM  pipeline=off  dbl_ovrd=off  block_type=cmult
  Delay1 : xbsIndex_r4/Delay  rst=off  infoeditControl=Selection of Reset will increase slice count due to use of real FFs and instead of SRLs  en=off  latency=1  reg_retiming=off  dbl_ovrd=off  block_type=delay
  Delay2 : xbsIndex_r4/Delay  rst=off  infoeditControl=Selection of Reset will increase slice count due to use of real FFs and instead of SRLs  en=off  latency=1  reg_retiming=off  dbl_ovrd=off  block_type=delay
  Delay3 : xbsIndex_r4/Delay  rst=off  infoeditControl=Selection of Reset will increase slice count due to use of real FFs and instead of SRLs  en=off  latency=1  reg_retiming=off  dbl_ovrd=off  block_type=delay
  Out1 : Outport
  wires:
  Delay1/1 -> CMult2/1, Delay2/1
  AddSub2/1 -> AddSub3/1
  Delay2/1 -> CMult1/1, Delay3/1
  CMult2/1 -> AddSub1/2
  Delay3/1 -> CMult3/1
  AddSub1/1 -> AddSub3/2
  In1/1 -> CMult4/1, Delay1/1
  CMult3/1 -> AddSub2/2
  AddSub3/1 -> Out1/1
  CMult4/1 -> AddSub1/1
  CMult1/1 -> AddSub2/1

== system exampleModel_bus_axi_w_4ptavg/example/dsp/Cav1/Subsystem/freq_err ==
  note: find ratio with NCO
  note: 2*pi*dt
  note: pi*(scaled_phi))
  note: w = d_phi/dt = (pi*(scaled_phi))/dt
  note: f=w/(2*pi)
  note: window for start/stop evaluating the phase
  raw_phase : Inport
  window : Inport  Port=2
  reset : Inport  Port=3
  AddSub : xbsIndex_r4/AddSub  mode=Addition  use_carryin=off  use_carryout=off  en=on  latency=1  precision=User Defined  arith_type="Signed  (2's comp)"  n_bits=64  bin_pt=32  quantization=Truncate  overflow=Saturate  use_behavioral_HDL=off  hw_selection=Fabric  pipelined=off  dbl_ovrd=off  block_type=addsub
  Constant1 : xbsIndex_r4/Constant  const=-Fsig  gui_display_data_type=Fixed-point  arith_type=Signed (2's comp)  n_bits=26  bin_pt=0  preci_type=Single  exp_width=8  frac_width=24  explicit_period=off  period=1  equ=P=C  opselect=C  inp2=PCIN>>17  opr=+  inp1=P  carry=CIN  dbl_ovrd=off  block_type=constant
  Constant8 : xbsIndex_r4/Constant  const=-Fsig  gui_display_data_type=Fixed-point  arith_type=Signed (2's comp)  n_bits=26  bin_pt=0  preci_type=Single  exp_width=8  frac_width=24  explicit_period=off  period=1  equ=P=C  opselect=C  inp2=PCIN>>17  opr=+  inp1=P  carry=CIN  dbl_ovrd=off  block_type=constant
  Convert : xbsIndex_r4/Convert  gui_display_data_type=Fixed-point  arith_type="Signed  (2's comp)"  n_bits=32  bin_pt=32  float_type=Single  exp_bits=8  fraction_bits=24  quantization=Truncate  overflow=Saturate  en=off  latency=1  pipeline=off  dbl_ovrd=off  block_type=convert
  Convert1 : xbsIndex_r4/Convert  gui_display_data_type=Fixed-point  arith_type="Signed  (2's comp)"  n_bits=32  bin_pt=32  float_type=Single  exp_bits=8  fraction_bits=24  quantization=Truncate  overflow=Saturate  en=off  latency=1  pipeline=off  dbl_ovrd=off  block_type=convert
  Convert3 : xbsIndex_r4/Convert  gui_display_data_type=Boolean  arith_type=Boolean  n_bits=16  bin_pt=14  float_type=Single  exp_bits=8  fraction_bits=24  quantization=Truncate  overflow=Wrap  en=off  latency=1  pipeline=off  dbl_ovrd=off  block_type=convert
  Delay : Delay  DelayLength=3  InitialCondition=0
  Delay1 : Delay  DelayLength=3  InitialCondition=0
  Delay2 : Delay  DelayLength=3  InitialCondition=0
  Delay3 : xbsIndex_r4/Delay  rst=off  infoeditControl=Selection of Reset will increase slice count due to use of real FFs and instead of SRLs  en=off  latency=10  reg_retiming=off  dbl_ovrd=off  block_type=delay
  Delay4 : xbsIndex_r4/Delay  rst=off  infoeditControl=Selection of Reset will increase slice count due to use of real FFs and instead of SRLs  en=off  latency=1  reg_retiming=off  dbl_ovrd=off  block_type=delay
  Delay5 : xbsIndex_r4/Delay  rst=off  infoeditControl=Selection of Reset will increase slice count due to use of real FFs and instead of SRLs  en=off  latency=1  reg_retiming=off  dbl_ovrd=off  block_type=delay
  Display1 : Display
  Display6 : Display
  Display8 : Display
  Divide : xbsIndex_r4/Divide  flow_control=NonBlocking  axi_optimize_goal=Resources  algorithm_type=Radix2  infoedit1=Specify output fraction-width for Fixed-point division.  fractional_width=31  infoedit2=Specify latency for Floating-point division.  latency=1  rate=1  has_a_tlast=off  has_a_tuser=off  has_b_tlast=off  has_b_tuser=off  en=off  has_result_tready=off  result_tlast_behv=Pass_A_TLAST  has_underflow=off  has_overflow=off  has_invalid_op=off  has_divide_by_zero=off  fpo_op_type=mergeddivide  block_type=divide
      settings: infoedit=Blocking: Wait for data on all inputs, allow back-pressure.<br>NonBlocking: operate every cycle in which all inputs are valid, no back-pressure.
  Divide1 : xbsIndex_r4/Divide  flow_control=NonBlocking  axi_optimize_goal=Resources  algorithm_type=Radix2  infoedit1=Specify output fraction-width for Fixed-point division.  fractional_width=33  infoedit2=Specify latency for Floating-point division.  latency=1  rate=1  has_a_tlast=off  has_a_tuser=off  has_b_tlast=off  has_b_tuser=off  en=off  has_result_tready=off  result_tlast_behv=Pass_A_TLAST  has_underflow=off  has_overflow=off  has_invalid_op=off  has_divide_by_zero=off  fpo_op_type=mergeddivide  block_type=divide
      settings: infoedit=Blocking: Wait for data on all inputs, allow back-pressure.<br>NonBlocking: operate every cycle in which all inputs are valid, no back-pressure.
  Divide2 : xbsIndex_r4/Divide  flow_control=NonBlocking  axi_optimize_goal=Resources  algorithm_type=Radix2  infoedit1=Specify output fraction-width for Fixed-point division.  fractional_width=33  infoedit2=Specify latency for Floating-point division.  latency=1  rate=1  has_a_tlast=off  has_a_tuser=off  has_b_tlast=off  has_b_tuser=off  en=off  has_result_tready=off  result_tlast_behv=Pass_A_TLAST  has_underflow=off  has_overflow=off  has_invalid_op=off  has_divide_by_zero=off  fpo_op_type=mergeddivide  block_type=divide
      settings: infoedit=Blocking: Wait for data on all inputs, allow back-pressure.<br>NonBlocking: operate every cycle in which all inputs are valid, no back-pressure.
  Down Sample : xbsIndex_r4/Down Sample  sample_ratio=12  sample_phase="Last Value of Frame  (most efficient)"  en=off  rst=off  latency=1  dbl_ovrd=off  block_type=dsamp
  Down Sample1 : xbsIndex_r4/Down Sample  sample_ratio=12  sample_phase="Last Value of Frame  (most efficient)"  en=off  rst=off  latency=1  dbl_ovrd=off  block_type=dsamp
  Down Sample8 : xbsIndex_r4/Down Sample  sample_ratio=12  sample_phase="Last Value of Frame  (most efficient)"  en=off  rst=off  latency=1  dbl_ovrd=off  block_type=dsamp
  Gateway Out{1..9,11,19..20} (12 alike) : xbsIndex_r4/Gateway Out  inherit_from_input=off  hdl_port=on  rows=1  columns=1  UseAsDAC=off  DACChannel='1'  interface=None  automatic_assignment=on  address_offset=hex2dec('00')  intf_name=''  intf_description=''  timing_constraint=None  locs_specified=off  LOCs={}  io_standard={}  block_type=gatewayout
  Inverter : xbsIndex_r4/Inverter  en=off  latency=1  dbl_ovrd=off  block_type=inv
  Logical1 : xbsIndex_r4/Logical  logical_function=AND  inputs=2  en=off  latency=1  precision=User Defined  arith_type=Boolean  n_bits=1  bin_pt=0  align_bp=on  dbl_ovrd=off  block_type=logical
  Mult3 : xbsIndex_r4/Mult  precision=User Defined  arith_type="Signed  (2's comp)"  n_bits=33  bin_pt=30  quantization=Truncate  overflow=Wrap  en=off  latency=3  use_behavioral_HDL=off  opt=Speed  use_embedded=on  optimum_pipeline=off  pipeline=on  dbl_ovrd=off  use_rpm=on  placement_style=Triangular  block_type=mult
  Register : xbsIndex_r4/Register  init=0  rst=on  en=on  dbl_ovrd=off  block_type=register
  Scope1 : Scope  NumInputPorts=2
  Scope2 : Scope  NumInputPorts=3
  Scope3 : Scope  NumInputPorts=3
  Scope4 : Scope  NumInputPorts=3
  delta_phi : Subsystem
  delta_t : Subsystem
  hi_bit_phi : Scope  NumInputPorts=4
  NCO_err : Outport
  tag scope: sim_f_err=global, testa=global
  wires:
  delta_t/1(dt) -> Divide/2
  delta_phi/1(d_phi) -> Divide/1
  reset/1 -> Convert3/1
  Gateway Out11/1 -> Scope2/2, Display8/1
  Gateway Out8/1 -> [sim_f_err], Scope2/1, Display6/1
  Gateway Out20/1 -> Delay1/1
  Convert3/1 -> delta_t/2(reset), delta_phi/3(reset)
  Gateway Out19/1 -> hi_bit_phi/2
  window/1 -> Gateway Out20/1, delta_t/1(window), delta_phi/2(window), Mult3/1
  Mult3/1 -> delta_phi/1(phase), Gateway Out19/1
  Constant8/1 -> Divide1/2
  Down Sample/1 -> Convert/1
  Divide1/1 -> Down Sample/1
  Gateway Out1/1 -> Scope1/2
  Gateway Out2/1 -> Scope1/1
  Gateway Out3/1 -> Delay/1
  Delay/1 -> hi_bit_phi/3
  [c1p2_pt_cntr] -> Gateway Out4/1
  Gateway Out4/1 -> Delay2/1
  Delay2/1 -> hi_bit_phi/4
  raw_phase/1 -> Gateway Out2/1, Gateway Out1/1, Mult3/2, Gateway Out3/1
  Delay1/1 -> Scope2/3, hi_bit_phi/1
  Convert/1 -> NCO_err/1, Gateway Out11/1
  delta_phi/2(val_latched) -> Delay3/1
  Logical1/1 -> Register/3, Delay5/1, Delay4/1, Gateway Out6/1
  Inverter/1 -> Logical1/1
  Delay3/1 -> Inverter/1, Logical1/2
  Gateway Out7/1 -> Display1/1, Scope3/1
  Gateway Out5/1 -> Scope3/2
  Gateway Out6/1 -> Scope3/3
  Divide/1 -> Down Sample8/1, Gateway Out8/1, Divide1/1
  Register/1 -> Gateway Out5/1, AddSub/1
  Delay5/1 -> Register/2
  Down Sample8/1 -> Register/1
  Delay4/1 -> AddSub/3
  Down Sample1/1 -> Convert1/1
  AddSub/1 -> Gateway Out9/1, Divide2/1, Gateway Out7/1, AddSub/2
  Divide2/1 -> Down Sample1/1
  Constant1/1 -> Divide2/2
  Gateway Out9/1 -> Scope4/1
  Convert1/1 -> [testa]

== system exampleModel_bus_axi_w_4ptavg/example/dsp/Cav1/Subsystem10/posedge_pulse ==
  In1 : Inport
  Inverter1 : xbsIndex_r4/Inverter  en=off  latency=1  dbl_ovrd=off  block_type=inv
  Logical : xbsIndex_r4/Logical  logical_function=AND  inputs=2  en=off  latency=1  precision=Full  arith_type=Unsigned  n_bits=16  bin_pt=0  align_bp=on  dbl_ovrd=off  block_type=logical
  Out1 : Outport
  wires:
  In1/1 -> Logical/1, Inverter1/1
  Logical/1 -> Out1/1
  Inverter1/1 -> Logical/2

== system exampleModel_bus_axi_w_4ptavg/example/dsp/Cav1/Subsystem11/posedge_pulse ==
  In1 : Inport
  Inverter1 : xbsIndex_r4/Inverter  en=off  latency=1  dbl_ovrd=off  block_type=inv
  Logical : xbsIndex_r4/Logical  logical_function=AND  inputs=2  en=off  latency=1  precision=Full  arith_type=Unsigned  n_bits=16  bin_pt=0  align_bp=on  dbl_ovrd=off  block_type=logical
  Out1 : Outport
  wires:
  Inverter1/1 -> Logical/2
  Logical/1 -> Out1/1
  In1/1 -> Inverter1/1, Logical/1

== system exampleModel_bus_axi_w_4ptavg/example/dsp/Cav1/Subsystem12/posedge_pulse ==
  In1 : Inport
  Inverter1 : xbsIndex_r4/Inverter  en=off  latency=1  dbl_ovrd=off  block_type=inv
  Logical : xbsIndex_r4/Logical  logical_function=AND  inputs=2  en=off  latency=1  precision=Full  arith_type=Unsigned  n_bits=16  bin_pt=0  align_bp=on  dbl_ovrd=off  block_type=logical
  Out1 : Outport
  wires:
  In1/1 -> Logical/1, Inverter1/1
  Logical/1 -> Out1/1
  Inverter1/1 -> Logical/2

== system exampleModel_bus_axi_w_4ptavg/example/dsp/Cav1/Subsystem13/posedge_pulse ==
  In1 : Inport
  Inverter1 : xbsIndex_r4/Inverter  en=off  latency=1  dbl_ovrd=off  block_type=inv
  Logical : xbsIndex_r4/Logical  logical_function=AND  inputs=2  en=off  latency=1  precision=Full  arith_type=Unsigned  n_bits=16  bin_pt=0  align_bp=on  dbl_ovrd=off  block_type=logical
  Out1 : Outport
  wires:
  Inverter1/1 -> Logical/2
  Logical/1 -> Out1/1
  In1/1 -> Inverter1/1, Logical/1

== system exampleModel_bus_axi_w_4ptavg/example/dsp/Cav1/Subsystem4/posedge_pulse ==
  In1 : Inport
  Inverter1 : xbsIndex_r4/Inverter  en=off  latency=1  dbl_ovrd=off  block_type=inv
  Logical : xbsIndex_r4/Logical  logical_function=AND  inputs=2  en=off  latency=1  precision=Full  arith_type=Unsigned  n_bits=16  bin_pt=0  align_bp=on  dbl_ovrd=off  block_type=logical
  Out1 : Outport
  wires:
  Inverter1/1 -> Logical/2
  Logical/1 -> Out1/1
  In1/1 -> Inverter1/1, Logical/1

== system exampleModel_bus_axi_w_4ptavg/example/dsp/Cav1/Subsystem5/posedge_pulse ==
  In1 : Inport
  Inverter1 : xbsIndex_r4/Inverter  en=off  latency=1  dbl_ovrd=off  block_type=inv
  Logical : xbsIndex_r4/Logical  logical_function=AND  inputs=2  en=off  latency=1  precision=Full  arith_type=Unsigned  n_bits=16  bin_pt=0  align_bp=on  dbl_ovrd=off  block_type=logical
  Out1 : Outport
  wires:
  In1/1 -> Logical/1, Inverter1/1
  Logical/1 -> Out1/1
  Inverter1/1 -> Logical/2

== system exampleModel_bus_axi_w_4ptavg/example/dsp/Cav1/Subsystem6/posedge_pulse ==
  In1 : Inport
  Inverter1 : xbsIndex_r4/Inverter  en=off  latency=1  dbl_ovrd=off  block_type=inv
  Logical : xbsIndex_r4/Logical  logical_function=AND  inputs=2  en=off  latency=1  precision=Full  arith_type=Unsigned  n_bits=16  bin_pt=0  align_bp=on  dbl_ovrd=off  block_type=logical
  Out1 : Outport
  wires:
  In1/1 -> Logical/1, Inverter1/1
  Logical/1 -> Out1/1
  Inverter1/1 -> Logical/2

== system exampleModel_bus_axi_w_4ptavg/example/dsp/Cav1/Subsystem7/posedge_pulse ==
  In1 : Inport
  Inverter1 : xbsIndex_r4/Inverter  en=off  latency=1  dbl_ovrd=off  block_type=inv
  Logical : xbsIndex_r4/Logical  logical_function=AND  inputs=2  en=off  latency=1  precision=Full  arith_type=Unsigned  n_bits=16  bin_pt=0  align_bp=on  dbl_ovrd=off  block_type=logical
  Out1 : Outport
  wires:
  Inverter1/1 -> Logical/2
  Logical/1 -> Out1/1
  In1/1 -> Inverter1/1, Logical/1

== system exampleModel_bus_axi_w_4ptavg/example/dsp/Cav1/Subsystem8/posedge_pulse ==
  In1 : Inport
  Inverter1 : xbsIndex_r4/Inverter  en=off  latency=1  dbl_ovrd=off  block_type=inv
  Logical : xbsIndex_r4/Logical  logical_function=AND  inputs=2  en=off  latency=1  precision=Full  arith_type=Unsigned  n_bits=16  bin_pt=0  align_bp=on  dbl_ovrd=off  block_type=logical
  Out1 : Outport
  wires:
  In1/1 -> Logical/1, Inverter1/1
  Logical/1 -> Out1/1
  Inverter1/1 -> Logical/2
